simulink model "PID_Controller_CodeGen_March9_2023a"  (R2023a)
settings: Solver=VariableStepAuto  StartTime=0.0  StopTime=10.0  RelTol=1e-3
undefined symbols (not defined in the file): Drive
libraries: robotlib x4, slpidlib x1
settings Model: Creator=abbas  LastModifiedBy=abbas

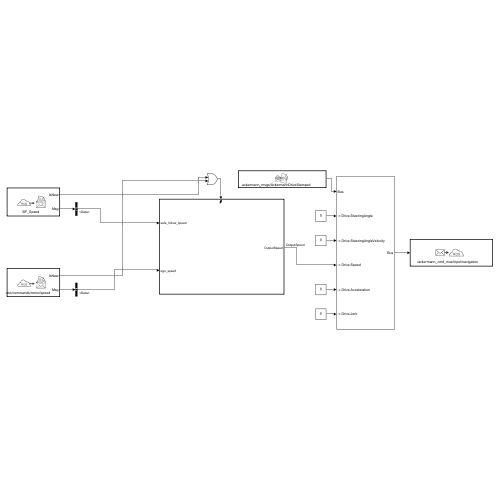
[thumbnail: Simulink's stored preview of the top-level diagram]
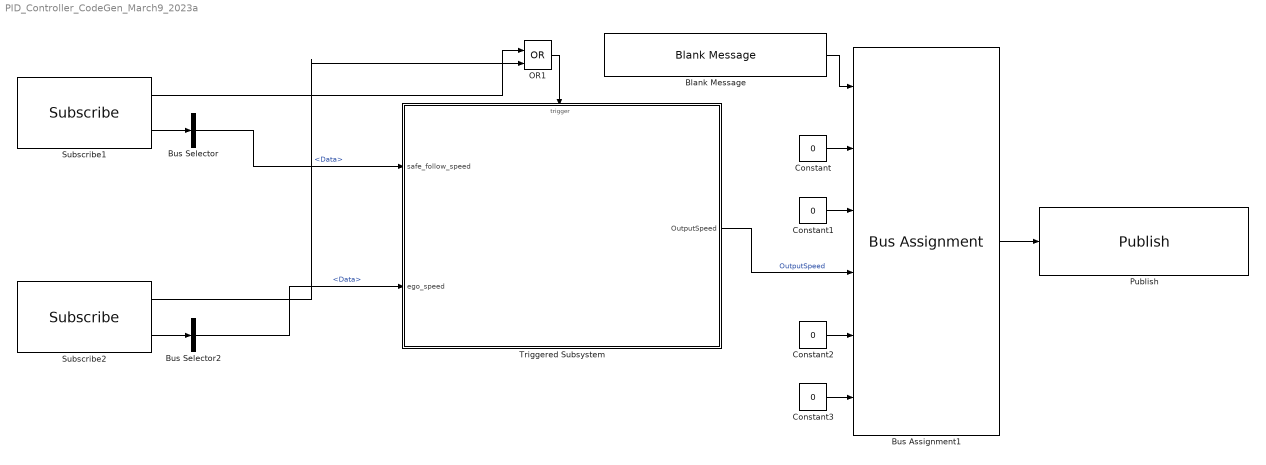
== system PID_Controller_CodeGen_March9_2023a ==
  Blank Message : robotlib/Blank Message  messageClass=Message  entityType=ackermann_msgs/AckermannDriveStamped  messageType=ackermann_msgs/AckermannDriveStamped  SampleTime=inf  legacyBusStruct=off
  Bus Assignment1 : BusAssignment  AssignedSignals=Drive.SteeringAngle,Drive.SteeringAngleVelocity,Drive.Speed,Drive.Acceleration,Drive.Jerk
  Bus Selector : BusSelector  OutputSignals=Data
  Bus Selector2 : BusSelector  OutputSignals=Data
  Constant{,1..3} (4 alike) : Constant  Value=0
  OR1 : Logic  Operator=OR  IconShape=distinctive  AllPortsSameDT=off  OutDataTypeStr=boolean
  Publish : robotlib/Publish  topicSource=Specify your own  topic=/ackermann_cmd_mux/input/navigation  messageType=ackermann_msgs/AckermannDriveStamped  legacyBusStruct=off  messageQueueLength=1
  Subscribe1 : robotlib/Subscribe  topicSource=Specify your own  topic=/SF_Speed  messageType=std_msgs/Float32  SampleTime=-1  legacyBusStruct=off  messageQueueLength=1
  Subscribe2 : robotlib/Subscribe  topicSource=Specify your own  topic=/vesc/commands/motor/speed  messageType=std_msgs/Float64  SampleTime=-1  legacyBusStruct=off  messageQueueLength=1
  Triggered Subsystem : Subsystem  TreatAsAtomicUnit=on
  wires:
  Bus Selector2/1 -> Triggered Subsystem/2(ego_speed)  "<Data>"
  Subscribe2/1 -> OR1/2
  Triggered Subsystem/1(OutputSpeed) -> Bus Assignment1/4  "OutputSpeed"
  Blank Message/1 -> Bus Assignment1/1
  Constant3/1 -> Bus Assignment1/6
  Bus Assignment1/1 -> Publish/1
  Subscribe1/2 -> Bus Selector/1
  Constant2/1 -> Bus Assignment1/5
  Constant1/1 -> Bus Assignment1/3
  Bus Selector/1 -> Triggered Subsystem/1(safe_follow_speed)  "<Data>"
  OR1/1 -> Triggered Subsystem/Trigger
  Subscribe2/2 -> Bus Selector2/1
  Constant/1 -> Bus Assignment1/2
  Subscribe1/1 -> OR1/1

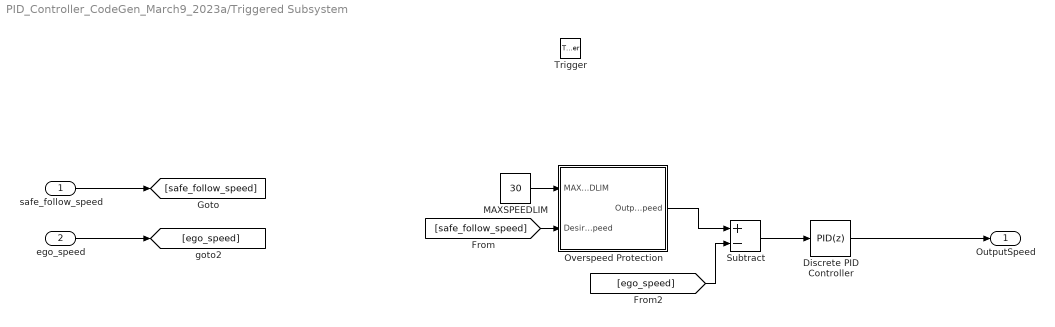
== system PID_Controller_CodeGen_March9_2023a/Triggered Subsystem ==
  safe_follow_speed : Inport
  ego_speed : Inport  Port=2
  Trigger : TriggerPort  VariantControl=(inherit)
  Discrete PID Controller : slpidlib/PID Controller  Controller=PID  Form=Parallel  TimeDomain=Discrete-time  UseExternalTs=off  SampleTime=0.1  IntegratorMethod=Forward Euler  FilterMethod=Forward Euler  ControllerParametersSource=internal  P=1.2  I=1  UseKiTs=on  D=0  N=100  UseFilter=on  TunerSelectOption=Frequency Response Based  InitialConditionSource=internal  InitialConditionForIntegrator=0  InitialConditionForFilter=0  DifferentiatorICPrevScaledInput=0  ExternalReset=none  TrackingMode=off  Kt=1  LimitOutput=off  SatLimitsSource=internal  UpperSaturationLimit=inf  LowerSaturationLimit=-inf  LinearizeAsGain=off  AntiWindupMode=none  Kb=1  LimitIntegrator=off  UpperIntegratorSaturationLimit=inf  LowerIntegratorSaturationLimit=-inf  POutMin=[]  POutMax=[]  IOutMin=[]  IOutMax=[]  DOutMin=[]  DOutMax=[]  NOutMin=[]  NOutMax=[]  SumOutMin=[]  SumOutMax=[]  SaturationOutMin=[]  SaturationOutMax=[]  PParamMin=[]  PParamMax=[]  IParamMin=[]  IParamMax=[]  DParamMin=[]  DParamMax=[]  NParamMin=[]  NParamMax=[]  KbParamMin=[]  KbParamMax=[]  KtParamMin=[]  KtParamMax=[]  KbOutMin=[]  KbOutMax=[]  KtOutMin=[]  KtOutMax=[]  IntegratorOutMin=[]  IntegratorOutMax=[]  FilterOutMin=[]  FilterOutMax=[]  SumI1OutMin=[]  SumI1OutMax=[]  SumI2OutMin=[]  SumI2OutMax=[]  SumI3OutMin=[]  SumI3OutMax=[]  SumI4OutMin=[]  SumI4OutMax=[]  SumDOutMin=[]  SumDOutMax=[]  DifferentiatorOutMin=[]  DifferentiatorOutMax=[]  FilterDiffOutCoefMin=[]  FilterDiffOutCoefMax=[]  ReciprocalOutMin=[]  ReciprocalOutMax=[]  SumDenOutMin=[]  SumDenOutMax=[]  SumNumOutMin=[]  SumNumOutMax=[]  DivideOutMin=[]  DivideOutMax=[]  UdiffTsProdOutMin=[]  UdiffTsProdOutMax=[]  NTsProdOutMin=[]  NTsProdOutMax=[]  UintegralTsProdOutMin=[]  UintegralTsProdOutMax=[]  UngainTsProdOutMin=[]  UngainTsProdOutMax=[]  ClampingZeroOutDataTypeStr=Inherit: Inherit via back propagation  ClampingZeroOutMin=[]  ClampingZeroOutMax=[]  FilterDenConstantOutDataTypeStr=Inherit: Inherit via back propagation  FilterDenConstantOutMin=[]  FilterDenConstantOutMax=[]  PCopyOutDataTypeStr=Inherit: Inherit via back propagation  PCopyOutMin=[]  PCopyOutMax=[]  NCopyOutDataTypeStr=Inherit: Inherit via back propagation  NCopyOutMin=[]  NCopyOutMax=[]  IntegratorContinuousStateAttributes=''  IntegratorStateMustResolveToSignalObject=off  IntegratorRTWStateStorageClass=Auto  FilterContinuousStateAttributes=''  FilterStateMustResolveToSignalObject=off  FilterRTWStateStorageClass=Auto  ParallelPVariant=InternalParameters  IdealPVariant=Disabled  IVariant=InternalParameters  DVariant=InternalParameters  IntegratorVariant=Discrete  SatVariant=Disabled  AWVariant=Passthrough  PCopyVariant=Disabled  TRVariant=Disabled  FdbkBlocksVariant=Forward  IdealPFdbkVariant=Disabled  SatFdbkVariant=Disabled  DerivativeFilterVariant=ForwardEulerFilter  NVariant=InternalParameters  NCopyVariant=Disabled  FilterICVariant=InternalICsFilter  IntegratorICVariant=InternalICs  ExternalResetVariant=Disabled  TRSumVariant=Passthrough  SumFdbkVariant=Disabled  SumVariant=Sum_PID  TsampFilterVariant=InternalTs  TsampNgainVariant=Passthrough  TsampIntegralVariant=Disabled_SignalSpec  ExternalSaturationOutDataTypeStr=Inherit: Same as second input
      settings: LibrarySourceBlock=simulink/Discrete/Discrete PID Controller
  MAXSPEEDLIM : Constant  Value=30
  Overspeed Protection : MATLAB Function  TreatAsAtomicUnit=on
  Subtract : Sum  Inputs=+-
  OutputSpeed : Outport
  wires:
  Discrete PID Controller/1 -> OutputSpeed/1
  Subtract/1 -> Discrete PID Controller/1
  safe_follow_speed/1 -> [safe_follow_speed]
  MAXSPEEDLIM/1 -> Overspeed Protection/1(MAXSPEEDLIM)
  Overspeed Protection/1(Output_Speed) -> Subtract/1
  [safe_follow_speed] -> Overspeed Protection/2(DesiredSpeed)
  ego_speed/1 -> [ego_speed]
  [ego_speed] -> Subtract/2

== matlab function PID_Controller_CodeGen_March9_2023a/Triggered Subsystem/Overspeed Protection ==
  data: MAXSPEEDLIM input; Output_Speed output; DesiredSpeed input
function Output_Speed  = fcn(MAXSPEEDLIM, DesiredSpeed)

if DesiredSpeed >= MAXSPEEDLIM
    Output_Speed = MAXSPEEDLIM;
elseif DesiredSpeed < 0
    Output_Speed = 0;
else 
    Output_Speed = DesiredSpeed;

end
